simulink model "OpenLoop_Controller"  (R2013b)
settings: Solver=FixedStepDiscrete  StartTime=0.0  StopTime=10  FixedStep=1/800  RelTol=1e-3
libraries: simulink x2
settings Model: Creator=m2memari  LastModifiedBy=m2memari
settings DataIOCC: SignalLoggingSaveFormat=ModelDataLogs
settings DebuggingCC: MultiTaskDSMMsg=warning  MultiTaskCondExecSysMsg=none
settings RTWCC: IncludeERTFirstTime=on

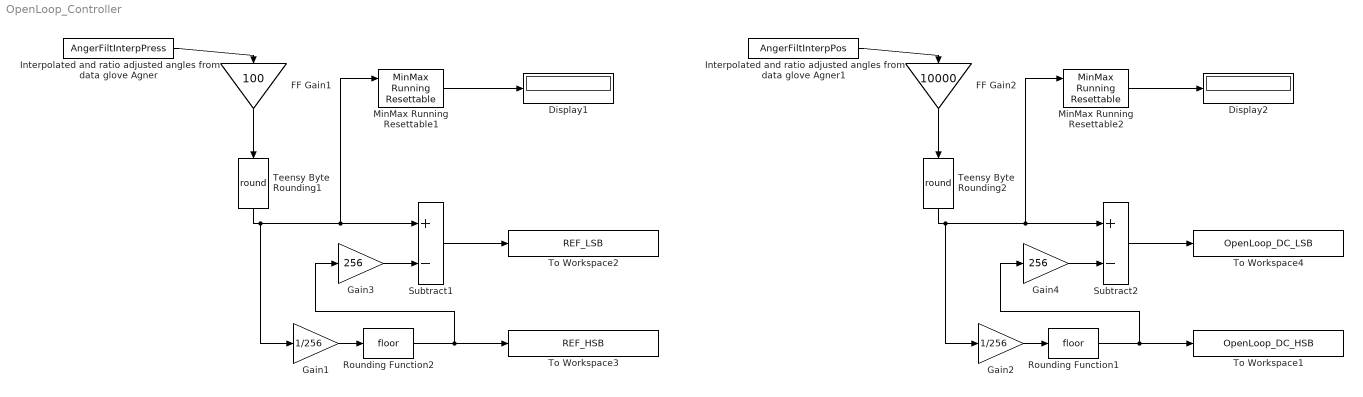
== system OpenLoop_Controller ==
  Display1 : Display
  Display2 : Display
  FF Gain1 : Gain  Gain=100
  FF Gain2 : Gain  Gain=10000
  Gain1 : Gain  Gain=1/256
  Gain2 : Gain  Gain=1/256
  Gain3 : Gain  Gain=256
  Gain4 : Gain  Gain=256
  Interpolated and ratio adjusted angles from data glove Agner : FromWorkspace  VariableName=AngerFiltInterpPress
  Interpolated and ratio adjusted angles from data glove Agner1 : FromWorkspace  VariableName=AngerFiltInterpPos
  MinMax Running Resettable1 : simulink/Math Operations/MinMax Running Resettable  Function=max  vinit=0.0
  MinMax Running Resettable2 : simulink/Math Operations/MinMax Running Resettable  Function=max  vinit=0.0
  Rounding Function1 : Rounding
  Rounding Function2 : Rounding
  Subtract1 : Sum  Inputs=+-
  Subtract2 : Sum  Inputs=+-
  Teensy Byte Rounding1 : Rounding  Operator=round
  Teensy Byte Rounding2 : Rounding  Operator=round
  To Workspace1 : ToWorkspace  VariableName=OpenLoop_DC_HSB  SampleTime=-1  SaveFormat=Timeseries
  To Workspace2 : ToWorkspace  VariableName=REF_LSB  SampleTime=-1  SaveFormat=Timeseries
  To Workspace3 : ToWorkspace  VariableName=REF_HSB  SampleTime=-1  SaveFormat=Timeseries
  To Workspace4 : ToWorkspace  VariableName=OpenLoop_DC_LSB  SampleTime=-1  SaveFormat=Timeseries
  wires:
  Gain1/1 -> Rounding Function2/1
  Rounding Function2/1 -> Gain3/1, To Workspace3/1
  Subtract1/1 -> To Workspace2/1
  Gain3/1 -> Subtract1/2
  FF Gain1/1 -> Teensy Byte Rounding1/1
  Teensy Byte Rounding1/1 -> MinMax Running Resettable1/1, Subtract1/1, Gain1/1
  MinMax Running Resettable1/1 -> Display1/1
  Interpolated and ratio adjusted angles from data glove Agner/1 -> FF Gain1/1
  Gain2/1 -> Rounding Function1/1
  Rounding Function1/1 -> To Workspace1/1, Gain4/1
  Subtract2/1 -> To Workspace4/1
  Gain4/1 -> Subtract2/2
  FF Gain2/1 -> Teensy Byte Rounding2/1
  Teensy Byte Rounding2/1 -> MinMax Running Resettable2/1, Subtract2/1, Gain2/1
  MinMax Running Resettable2/1 -> Display2/1
  Interpolated and ratio adjusted angles from data glove Agner1/1 -> FF Gain2/1
